simulink library "Nibble_Multiplexers_Lib"  (Simulink 8.7)
settings: Solver=ode45  StartTime=0.0  StopTime=10.0  RelTol=1e-3
libraries: Bit_Multiplexers_Lib x20, commutil2 x16
(part 1 of 2)
settings Model: Creator=uzivatel  LastModifiedBy=Jozko Mrkvicka

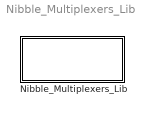
== system Nibble_Multiplexers_Lib ==
  Nibble_Multiplexers_Lib : Subsystem

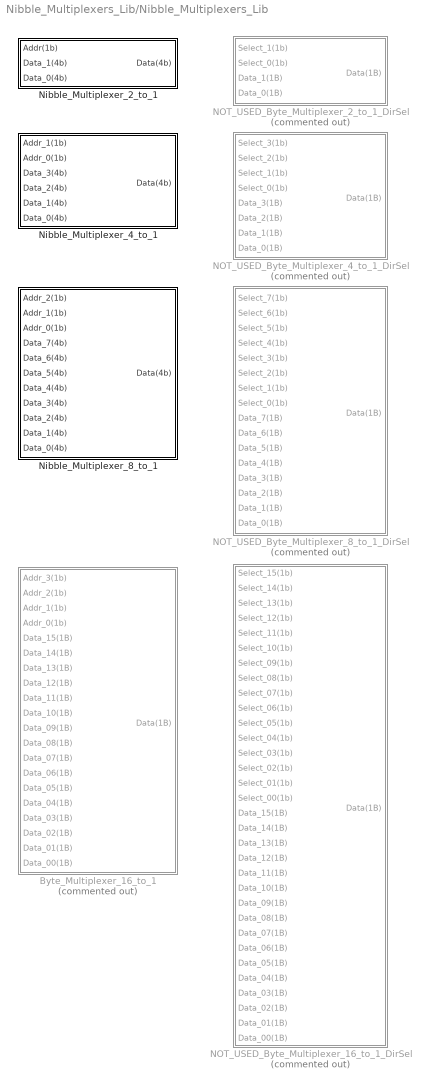
== system Nibble_Multiplexers_Lib/Nibble_Multiplexers_Lib ==
  Byte_Multiplexer_16_to_1 : Subsystem  Commented=on
  NOT_USED_Byte_Multiplexer_16_to_1_DirSel : Subsystem  Commented=on
  NOT_USED_Byte_Multiplexer_2_to_1_DirSel : Subsystem  Commented=on
  NOT_USED_Byte_Multiplexer_4_to_1_DirSel : Subsystem  Commented=on
  NOT_USED_Byte_Multiplexer_8_to_1_DirSel : Subsystem  Commented=on
  Nibble_Multiplexer_2_to_1 : Subsystem
  Nibble_Multiplexer_4_to_1 : Subsystem
  Nibble_Multiplexer_8_to_1 : Subsystem

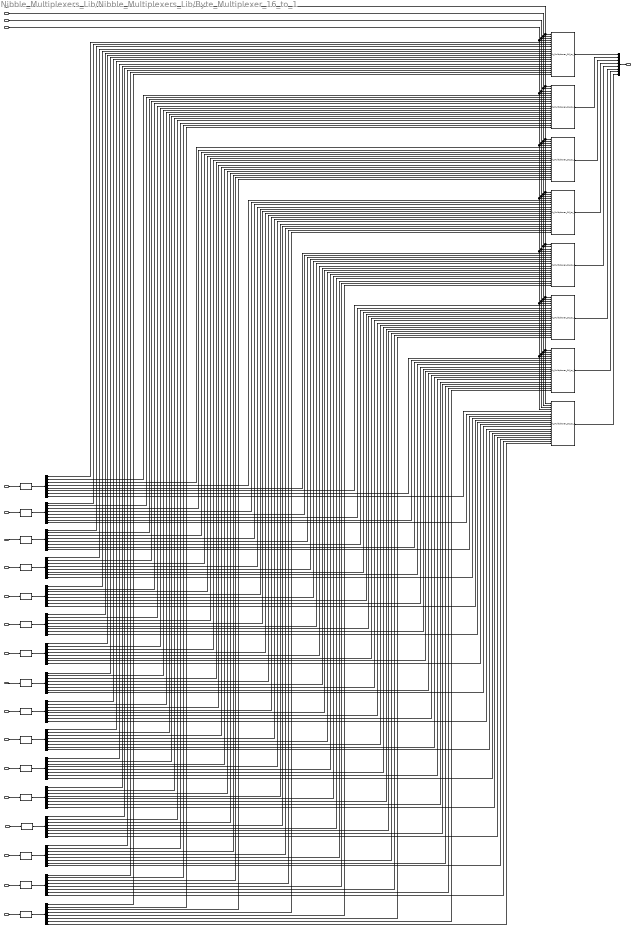
== system Nibble_Multiplexers_Lib/Nibble_Multiplexers_Lib/Byte_Multiplexer_16_to_1 ==
  Addr_3(1b) : Inport
  Addr_2(1b) : Inport  Port=2
  Addr_1(1b) : Inport  Port=3
  Addr_0(1b) : Inport  Port=4
  Data_15(1B) : Inport  Port=5
  Data_14(1B) : Inport  Port=6
  Data_13(1B) : Inport  Port=7
  Data_12(1B) : Inport  Port=8
  Data_11(1B) : Inport  Port=9
  Data_10(1B) : Inport  Port=10
  Data_09(1B) : Inport  Port=11
  Data_08(1B) : Inport  Port=12
  Data_07(1B) : Inport  Port=13
  Data_06(1B) : Inport  Port=14
  Data_05(1B) : Inport  Port=15
  Data_04(1B) : Inport  Port=16
  Data_03(1B) : Inport  Port=17
  Data_02(1B) : Inport  Port=18
  Data_01(1B) : Inport  Port=19
  Data_00(1B) : Inport  Port=20
  Bit_Multiplexer_16_to_1(Bit_0) : Bit_Multiplexers_Lib/Bit_Multiplexers_Lib/Bit_Multiplexer_16_to_1
  Bit_Multiplexer_16_to_1(Bit_1) : Bit_Multiplexers_Lib/Bit_Multiplexers_Lib/Bit_Multiplexer_16_to_1
  Bit_Multiplexer_16_to_1(Bit_2) : Bit_Multiplexers_Lib/Bit_Multiplexers_Lib/Bit_Multiplexer_16_to_1
  Bit_Multiplexer_16_to_1(Bit_3) : Bit_Multiplexers_Lib/Bit_Multiplexers_Lib/Bit_Multiplexer_16_to_1
  Bit_Multiplexer_16_to_1(Bit_4) : Bit_Multiplexers_Lib/Bit_Multiplexers_Lib/Bit_Multiplexer_16_to_1
  Bit_Multiplexer_16_to_1(Bit_5) : Bit_Multiplexers_Lib/Bit_Multiplexers_Lib/Bit_Multiplexer_16_to_1
  Bit_Multiplexer_16_to_1(Bit_6) : Bit_Multiplexers_Lib/Bit_Multiplexers_Lib/Bit_Multiplexer_16_to_1
  Bit_Multiplexer_16_to_1(Bit_7) : Bit_Multiplexers_Lib/Bit_Multiplexers_Lib/Bit_Multiplexer_16_to_1
  Bus Creator : BusCreator  Inputs=8
  Byte_{0..15} (16 alike) : Demux  Outputs=8
  Integer to Bit Converter{1..16} (16 alike) : commutil2/Integer to Bit Converter  nbits=8  signedInputValues=Unsigned  bitOrder=MSB first  outDtype=boolean
  Data(1B) : Outport
  wires:
  Integer to Bit Converter7/1 -> Byte_15/1
  Data_15(1B)/1 -> Integer to Bit Converter7/1
  Bus Creator/1 -> Data(1B)/1
  Addr_0(1b)/1 -> Bit_Multiplexer_16_to_1(Bit_5)/4, Bit_Multiplexer_16_to_1(Bit_0)/4, Bit_Multiplexer_16_to_1(Bit_1)/4, Bit_Multiplexer_16_to_1(Bit_2)/4, Bit_Multiplexer_16_to_1(Bit_3)/4, Bit_Multiplexer_16_to_1(Bit_4)/4, Bit_Multiplexer_16_to_1(Bit_6)/4, Bit_Multiplexer_16_to_1(Bit_7)/4
  Addr_1(1b)/1 -> Bit_Multiplexer_16_to_1(Bit_5)/3, Bit_Multiplexer_16_to_1(Bit_0)/3, Bit_Multiplexer_16_to_1(Bit_1)/3, Bit_Multiplexer_16_to_1(Bit_2)/3, Bit_Multiplexer_16_to_1(Bit_3)/3, Bit_Multiplexer_16_to_1(Bit_4)/3, Bit_Multiplexer_16_to_1(Bit_6)/3, Bit_Multiplexer_16_to_1(Bit_7)/3
  Addr_2(1b)/1 -> Bit_Multiplexer_16_to_1(Bit_6)/2, Bit_Multiplexer_16_to_1(Bit_5)/2, Bit_Multiplexer_16_to_1(Bit_4)/2, Bit_Multiplexer_16_to_1(Bit_2)/2, Bit_Multiplexer_16_to_1(Bit_1)/2, Bit_Multiplexer_16_to_1(Bit_0)/2, Bit_Multiplexer_16_to_1(Bit_3)/2, Bit_Multiplexer_16_to_1(Bit_7)/2
  Addr_3(1b)/1 -> Bit_Multiplexer_16_to_1(Bit_5)/1, Bit_Multiplexer_16_to_1(Bit_0)/1, Bit_Multiplexer_16_to_1(Bit_1)/1, Bit_Multiplexer_16_to_1(Bit_2)/1, Bit_Multiplexer_16_to_1(Bit_3)/1, Bit_Multiplexer_16_to_1(Bit_4)/1, Bit_Multiplexer_16_to_1(Bit_6)/1, Bit_Multiplexer_16_to_1(Bit_7)/1
  Bit_Multiplexer_16_to_1(Bit_4)/1 -> Bus Creator/4
  Bit_Multiplexer_16_to_1(Bit_5)/1 -> Bus Creator/3
  Bit_Multiplexer_16_to_1(Bit_6)/1 -> Bus Creator/2
  Bit_Multiplexer_16_to_1(Bit_7)/1 -> Bus Creator/1
  Bit_Multiplexer_16_to_1(Bit_3)/1 -> Bus Creator/5
  Bit_Multiplexer_16_to_1(Bit_2)/1 -> Bus Creator/6
  Bit_Multiplexer_16_to_1(Bit_1)/1 -> Bus Creator/7
  Bit_Multiplexer_16_to_1(Bit_0)/1 -> Bus Creator/8
  Integer to Bit Converter1/1 -> Byte_14/1
  Data_14(1B)/1 -> Integer to Bit Converter1/1
  Integer to Bit Converter2/1 -> Byte_13/1
  Data_13(1B)/1 -> Integer to Bit Converter2/1
  Integer to Bit Converter3/1 -> Byte_12/1
  Data_12(1B)/1 -> Integer to Bit Converter3/1
  Integer to Bit Converter4/1 -> Byte_11/1
  Data_11(1B)/1 -> Integer to Bit Converter4/1
  Integer to Bit Converter5/1 -> Byte_10/1
  Data_10(1B)/1 -> Integer to Bit Converter5/1
  Integer to Bit Converter6/1 -> Byte_9/1
  Data_09(1B)/1 -> Integer to Bit Converter6/1
  Integer to Bit Converter8/1 -> Byte_8/1
  Data_08(1B)/1 -> Integer to Bit Converter8/1
  Integer to Bit Converter9/1 -> Byte_7/1
  Data_07(1B)/1 -> Integer to Bit Converter9/1
  Integer to Bit Converter10/1 -> Byte_6/1
  Data_06(1B)/1 -> Integer to Bit Converter10/1
  Integer to Bit Converter11/1 -> Byte_5/1
  Data_05(1B)/1 -> Integer to Bit Converter11/1
  Integer to Bit Converter12/1 -> Byte_4/1
  Data_04(1B)/1 -> Integer to Bit Converter12/1
  Integer to Bit Converter13/1 -> Byte_3/1
  Data_03(1B)/1 -> Integer to Bit Converter13/1
  Integer to Bit Converter14/1 -> Byte_2/1
  Data_02(1B)/1 -> Integer to Bit Converter14/1
  Integer to Bit Converter15/1 -> Byte_1/1
  Data_01(1B)/1 -> Integer to Bit Converter15/1
  Integer to Bit Converter16/1 -> Byte_0/1
  Data_00(1B)/1 -> Integer to Bit Converter16/1
  Byte_15/1 -> Bit_Multiplexer_16_to_1(Bit_7)/5
  Byte_14/1 -> Bit_Multiplexer_16_to_1(Bit_7)/6
  Byte_13/1 -> Bit_Multiplexer_16_to_1(Bit_7)/7
  Byte_12/1 -> Bit_Multiplexer_16_to_1(Bit_7)/8
  Byte_11/1 -> Bit_Multiplexer_16_to_1(Bit_7)/9
  Byte_10/1 -> Bit_Multiplexer_16_to_1(Bit_7)/10
  Byte_9/1 -> Bit_Multiplexer_16_to_1(Bit_7)/11
  Byte_8/1 -> Bit_Multiplexer_16_to_1(Bit_7)/12
  Byte_7/1 -> Bit_Multiplexer_16_to_1(Bit_7)/13
  Byte_6/1 -> Bit_Multiplexer_16_to_1(Bit_7)/14
  Byte_5/1 -> Bit_Multiplexer_16_to_1(Bit_7)/15
  Byte_4/1 -> Bit_Multiplexer_16_to_1(Bit_7)/16
  Byte_3/1 -> Bit_Multiplexer_16_to_1(Bit_7)/17
  Byte_2/1 -> Bit_Multiplexer_16_to_1(Bit_7)/18
  Byte_1/1 -> Bit_Multiplexer_16_to_1(Bit_7)/19
  Byte_0/1 -> Bit_Multiplexer_16_to_1(Bit_7)/20
  Byte_15/2 -> Bit_Multiplexer_16_to_1(Bit_6)/5
  Byte_14/2 -> Bit_Multiplexer_16_to_1(Bit_6)/6
  Byte_13/2 -> Bit_Multiplexer_16_to_1(Bit_6)/7
  Byte_12/2 -> Bit_Multiplexer_16_to_1(Bit_6)/8
  Byte_11/2 -> Bit_Multiplexer_16_to_1(Bit_6)/9
  Byte_10/2 -> Bit_Multiplexer_16_to_1(Bit_6)/10
  Byte_9/2 -> Bit_Multiplexer_16_to_1(Bit_6)/11
  Byte_8/2 -> Bit_Multiplexer_16_to_1(Bit_6)/12
  Byte_7/2 -> Bit_Multiplexer_16_to_1(Bit_6)/13
  Byte_6/2 -> Bit_Multiplexer_16_to_1(Bit_6)/14
  Byte_5/2 -> Bit_Multiplexer_16_to_1(Bit_6)/15
  Byte_4/2 -> Bit_Multiplexer_16_to_1(Bit_6)/16
  Byte_3/2 -> Bit_Multiplexer_16_to_1(Bit_6)/17
  Byte_2/2 -> Bit_Multiplexer_16_to_1(Bit_6)/18
  Byte_1/2 -> Bit_Multiplexer_16_to_1(Bit_6)/19
  Byte_0/2 -> Bit_Multiplexer_16_to_1(Bit_6)/20
  Byte_15/3 -> Bit_Multiplexer_16_to_1(Bit_5)/5
  Byte_14/3 -> Bit_Multiplexer_16_to_1(Bit_5)/6
  Byte_13/3 -> Bit_Multiplexer_16_to_1(Bit_5)/7
  Byte_12/3 -> Bit_Multiplexer_16_to_1(Bit_5)/8
  Byte_11/3 -> Bit_Multiplexer_16_to_1(Bit_5)/9
  Byte_10/3 -> Bit_Multiplexer_16_to_1(Bit_5)/10
  Byte_9/3 -> Bit_Multiplexer_16_to_1(Bit_5)/11
  Byte_8/3 -> Bit_Multiplexer_16_to_1(Bit_5)/12
  Byte_7/3 -> Bit_Multiplexer_16_to_1(Bit_5)/13
  Byte_6/3 -> Bit_Multiplexer_16_to_1(Bit_5)/14
  Byte_5/3 -> Bit_Multiplexer_16_to_1(Bit_5)/15
  Byte_4/3 -> Bit_Multiplexer_16_to_1(Bit_5)/16
  Byte_3/3 -> Bit_Multiplexer_16_to_1(Bit_5)/17
  Byte_2/3 -> Bit_Multiplexer_16_to_1(Bit_5)/18
  Byte_1/3 -> Bit_Multiplexer_16_to_1(Bit_5)/19
  Byte_0/3 -> Bit_Multiplexer_16_to_1(Bit_5)/20
  Byte_15/4 -> Bit_Multiplexer_16_to_1(Bit_4)/5
  Byte_14/4 -> Bit_Multiplexer_16_to_1(Bit_4)/6
  Byte_13/4 -> Bit_Multiplexer_16_to_1(Bit_4)/7
  Byte_12/4 -> Bit_Multiplexer_16_to_1(Bit_4)/8
  Byte_11/4 -> Bit_Multiplexer_16_to_1(Bit_4)/9
  Byte_10/4 -> Bit_Multiplexer_16_to_1(Bit_4)/10
  Byte_9/4 -> Bit_Multiplexer_16_to_1(Bit_4)/11
  Byte_8/4 -> Bit_Multiplexer_16_to_1(Bit_4)/12
  Byte_7/4 -> Bit_Multiplexer_16_to_1(Bit_4)/13
  Byte_6/4 -> Bit_Multiplexer_16_to_1(Bit_4)/14
  Byte_5/4 -> Bit_Multiplexer_16_to_1(Bit_4)/15
  Byte_4/4 -> Bit_Multiplexer_16_to_1(Bit_4)/16
  Byte_3/4 -> Bit_Multiplexer_16_to_1(Bit_4)/17
  Byte_2/4 -> Bit_Multiplexer_16_to_1(Bit_4)/18
  Byte_1/4 -> Bit_Multiplexer_16_to_1(Bit_4)/19
  Byte_0/4 -> Bit_Multiplexer_16_to_1(Bit_4)/20
  Byte_15/5 -> Bit_Multiplexer_16_to_1(Bit_3)/5
  Byte_14/5 -> Bit_Multiplexer_16_to_1(Bit_3)/6
  Byte_13/5 -> Bit_Multiplexer_16_to_1(Bit_3)/7
  Byte_12/5 -> Bit_Multiplexer_16_to_1(Bit_3)/8
  Byte_11/5 -> Bit_Multiplexer_16_to_1(Bit_3)/9
  Byte_10/5 -> Bit_Multiplexer_16_to_1(Bit_3)/10
  Byte_9/5 -> Bit_Multiplexer_16_to_1(Bit_3)/11
  Byte_8/5 -> Bit_Multiplexer_16_to_1(Bit_3)/12
  Byte_7/5 -> Bit_Multiplexer_16_to_1(Bit_3)/13
  Byte_6/5 -> Bit_Multiplexer_16_to_1(Bit_3)/14
  Byte_5/5 -> Bit_Multiplexer_16_to_1(Bit_3)/15
  Byte_4/5 -> Bit_Multiplexer_16_to_1(Bit_3)/16
  Byte_3/5 -> Bit_Multiplexer_16_to_1(Bit_3)/17
  Byte_2/5 -> Bit_Multiplexer_16_to_1(Bit_3)/18
  Byte_1/5 -> Bit_Multiplexer_16_to_1(Bit_3)/19
  Byte_0/5 -> Bit_Multiplexer_16_to_1(Bit_3)/20
  Byte_15/6 -> Bit_Multiplexer_16_to_1(Bit_2)/5
  Byte_14/6 -> Bit_Multiplexer_16_to_1(Bit_2)/6
  Byte_13/6 -> Bit_Multiplexer_16_to_1(Bit_2)/7
  Byte_12/6 -> Bit_Multiplexer_16_to_1(Bit_2)/8
  Byte_11/6 -> Bit_Multiplexer_16_to_1(Bit_2)/9
  Byte_10/6 -> Bit_Multiplexer_16_to_1(Bit_2)/10
  Byte_9/6 -> Bit_Multiplexer_16_to_1(Bit_2)/11
  Byte_8/6 -> Bit_Multiplexer_16_to_1(Bit_2)/12
  Byte_7/6 -> Bit_Multiplexer_16_to_1(Bit_2)/13
  Byte_6/6 -> Bit_Multiplexer_16_to_1(Bit_2)/14
  Byte_5/6 -> Bit_Multiplexer_16_to_1(Bit_2)/15
  Byte_4/6 -> Bit_Multiplexer_16_to_1(Bit_2)/16
  Byte_3/6 -> Bit_Multiplexer_16_to_1(Bit_2)/17
  Byte_2/6 -> Bit_Multiplexer_16_to_1(Bit_2)/18
  Byte_1/6 -> Bit_Multiplexer_16_to_1(Bit_2)/19
  Byte_0/6 -> Bit_Multiplexer_16_to_1(Bit_2)/20
  Byte_15/7 -> Bit_Multiplexer_16_to_1(Bit_1)/5
  Byte_14/7 -> Bit_Multiplexer_16_to_1(Bit_1)/6
  Byte_13/7 -> Bit_Multiplexer_16_to_1(Bit_1)/7
  Byte_12/7 -> Bit_Multiplexer_16_to_1(Bit_1)/8
  Byte_11/7 -> Bit_Multiplexer_16_to_1(Bit_1)/9
  Byte_10/7 -> Bit_Multiplexer_16_to_1(Bit_1)/10
  Byte_9/7 -> Bit_Multiplexer_16_to_1(Bit_1)/11
  Byte_8/7 -> Bit_Multiplexer_16_to_1(Bit_1)/12
  Byte_7/7 -> Bit_Multiplexer_16_to_1(Bit_1)/13
  Byte_6/7 -> Bit_Multiplexer_16_to_1(Bit_1)/14
  Byte_5/7 -> Bit_Multiplexer_16_to_1(Bit_1)/15
  Byte_4/7 -> Bit_Multiplexer_16_to_1(Bit_1)/16
  Byte_3/7 -> Bit_Multiplexer_16_to_1(Bit_1)/17
  Byte_2/7 -> Bit_Multiplexer_16_to_1(Bit_1)/18
  Byte_1/7 -> Bit_Multiplexer_16_to_1(Bit_1)/19
  Byte_0/7 -> Bit_Multiplexer_16_to_1(Bit_1)/20
  Byte_15/8 -> Bit_Multiplexer_16_to_1(Bit_0)/5
  Byte_14/8 -> Bit_Multiplexer_16_to_1(Bit_0)/6
  Byte_13/8 -> Bit_Multiplexer_16_to_1(Bit_0)/7
  Byte_12/8 -> Bit_Multiplexer_16_to_1(Bit_0)/8
  Byte_11/8 -> Bit_Multiplexer_16_to_1(Bit_0)/9
  Byte_10/8 -> Bit_Multiplexer_16_to_1(Bit_0)/10
  Byte_9/8 -> Bit_Multiplexer_16_to_1(Bit_0)/11
  Byte_8/8 -> Bit_Multiplexer_16_to_1(Bit_0)/12
  Byte_7/8 -> Bit_Multiplexer_16_to_1(Bit_0)/13
  Byte_6/8 -> Bit_Multiplexer_16_to_1(Bit_0)/14
  Byte_5/8 -> Bit_Multiplexer_16_to_1(Bit_0)/15
  Byte_4/8 -> Bit_Multiplexer_16_to_1(Bit_0)/16
  Byte_3/8 -> Bit_Multiplexer_16_to_1(Bit_0)/17
  Byte_2/8 -> Bit_Multiplexer_16_to_1(Bit_0)/18
  Byte_1/8 -> Bit_Multiplexer_16_to_1(Bit_0)/19
  Byte_0/8 -> Bit_Multiplexer_16_to_1(Bit_0)/20

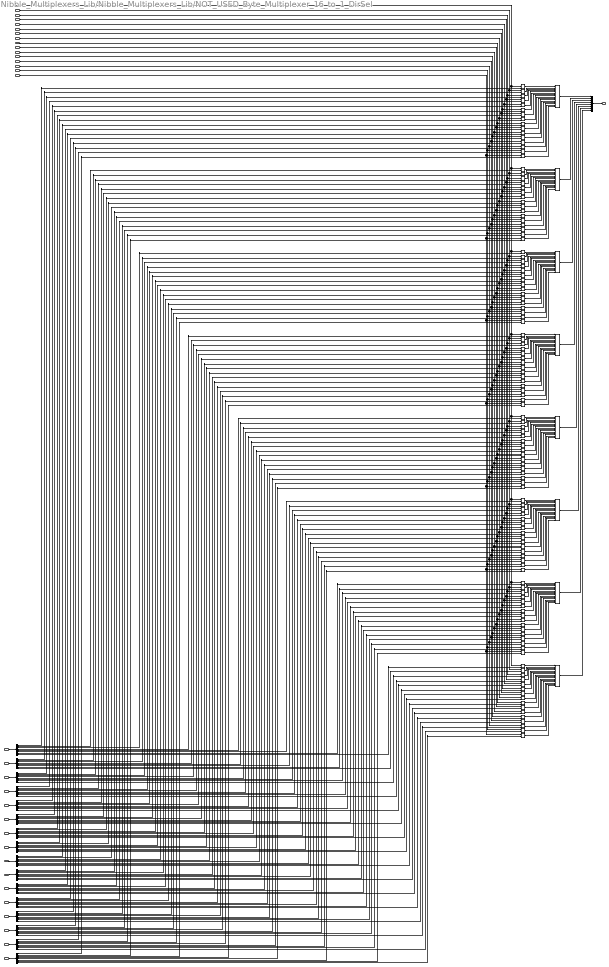
== system Nibble_Multiplexers_Lib/Nibble_Multiplexers_Lib/NOT_USED_Byte_Multiplexer_16_to_1_DirSel ==
  note: Bit_Multiplexer_16_to_1_DirSel(Bit_07)
  note: Bit_Multiplexer_16_to_1_DirSel(Bit_06)
  note: Bit_Multiplexer_16_to_1_DirSel(Bit_05)
  note: Bit_Multiplexer_16_to_1_DirSel(Bit_04)
  note: Bit_Multiplexer_16_to_1_DirSel(Bit_03)
  note: Bit_Multiplexer_16_to_1_DirSel(Bit_02)
  note: Bit_Multiplexer_16_to_1_DirSel(Bit_01)
  note: Bit_Multiplexer_16_to_1_DirSel(Bit_00)
  Select_15(1b) : Inport
  Select_14(1b) : Inport  Port=2
  Select_13(1b) : Inport  Port=3
  Select_12(1b) : Inport  Port=4
  Select_11(1b) : Inport  Port=5
  Select_10(1b) : Inport  Port=6
  Select_09(1b) : Inport  Port=7
  Select_08(1b) : Inport  Port=8
  Select_07(1b) : Inport  Port=9
  Select_06(1b) : Inport  Port=10
  Select_05(1b) : Inport  Port=11
  Select_04(1b) : Inport  Port=12
  Select_03(1b) : Inport  Port=13
  Select_02(1b) : Inport  Port=14
  Select_01(1b) : Inport  Port=15
  Select_00(1b) : Inport  Port=16
  Data_15(1B) : Inport  Port=17
  Data_14(1B) : Inport  Port=18
  Data_13(1B) : Inport  Port=19
  Data_12(1B) : Inport  Port=20
  Data_11(1B) : Inport  Port=21
  Data_10(1B) : Inport  Port=22
  Data_09(1B) : Inport  Port=23
  Data_08(1B) : Inport  Port=24
  Data_07(1B) : Inport  Port=25
  Data_06(1B) : Inport  Port=26
  Data_05(1B) : Inport  Port=27
  Data_04(1B) : Inport  Port=28
  Data_03(1B) : Inport  Port=29
  Data_02(1B) : Inport  Port=30
  Data_01(1B) : Inport  Port=31
  Data_00(1B) : Inport  Port=32
  Bus Creator : BusCreator  Inputs=8
  Bus Selector{1..16} (16 alike) : BusSelector  OutputSignals=signal1,signal2,signal3,signal4,signal5,signal6,signal7,signal8
  Logical Operator{137..151,153..168,170..185,187..202,204..219,221..236,238..253,255..270,272} (128 alike) : Logic  IconShape=distinctive  AllPortsSameDT=off  OutDataTypeStr=boolean
  Logical Operator{152,169,186,203,220,237,254,271} (8 alike) : Logic  Operator=OR  Inputs=16  IconShape=distinctive  OutDataTypeStr=boolean
  Data(1B) : Outport
  wires:
  Data_15(1B)/1 -> Bus Selector15/1
  Data_14(1B)/1 -> Bus Selector1/1
  Data_13(1B)/1 -> Bus Selector2/1
  Data_12(1B)/1 -> Bus Selector3/1
  Data_11(1B)/1 -> Bus Selector4/1
  Data_10(1B)/1 -> Bus Selector5/1
  Data_09(1B)/1 -> Bus Selector6/1
  Data_08(1B)/1 -> Bus Selector7/1
  Data_07(1B)/1 -> Bus Selector8/1
  Data_06(1B)/1 -> Bus Selector9/1
  Data_05(1B)/1 -> Bus Selector10/1
  Data_04(1B)/1 -> Bus Selector11/1
  Data_03(1B)/1 -> Bus Selector12/1
  Data_02(1B)/1 -> Bus Selector13/1
  Data_01(1B)/1 -> Bus Selector14/1
  Data_00(1B)/1 -> Bus Selector16/1
  Bus Creator/1 -> Data(1B)/1
  Bus Selector16/8 -> Logical Operator264/2  "<signal8>"
  Bus Selector14/8 -> Logical Operator263/2  "<signal8>"
  Bus Selector13/8 -> Logical Operator262/2  "<signal8>"
  Bus Selector12/8 -> Logical Operator261/2  "<signal8>"
  Bus Selector11/8 -> Logical Operator258/2  "<signal8>"
  Bus Selector10/8 -> Logical Operator257/2  "<signal8>"
  Bus Selector9/8 -> Logical Operator256/2  "<signal8>"
  Bus Selector8/8 -> Logical Operator272/2  "<signal8>"
  Bus Selector15/8 -> Logical Operator259/2  "<signal8>"
  Bus Selector1/8 -> Logical Operator260/2  "<signal8>"
  Bus Selector2/8 -> Logical Operator265/2  "<signal8>"
  Bus Selector3/8 -> Logical Operator266/2  "<signal8>"
  Bus Selector4/8 -> Logical Operator267/2  "<signal8>"
  Bus Selector5/8 -> Logical Operator268/2  "<signal8>"
  Bus Selector6/8 -> Logical Operator269/2  "<signal8>"
  Bus Selector7/8 -> Logical Operator270/2  "<signal8>"
  Bus Selector16/7 -> Logical Operator247/2  "<signal7>"
  Bus Selector14/7 -> Logical Operator246/2  "<signal7>"
  Bus Selector13/7 -> Logical Operator245/2  "<signal7>"
  Bus Selector12/7 -> Logical Operator244/2  "<signal7>"
  Bus Selector11/7 -> Logical Operator241/2  "<signal7>"
  Bus Selector10/7 -> Logical Operator240/2  "<signal7>"
  Bus Selector9/7 -> Logical Operator239/2  "<signal7>"
  Bus Selector8/7 -> Logical Operator255/2  "<signal7>"
  Bus Selector15/7 -> Logical Operator242/2  "<signal7>"
  Bus Selector1/7 -> Logical Operator243/2  "<signal7>"
  Bus Selector2/7 -> Logical Operator248/2  "<signal7>"
  Bus Selector3/7 -> Logical Operator249/2  "<signal7>"
  Bus Selector4/7 -> Logical Operator250/2  "<signal7>"
  Bus Selector5/7 -> Logical Operator251/2  "<signal7>"
  Bus Selector6/7 -> Logical Operator252/2  "<signal7>"
  Bus Selector7/7 -> Logical Operator253/2  "<signal7>"
  Bus Selector16/6 -> Logical Operator230/2  "<signal6>"
  Bus Selector14/6 -> Logical Operator229/2  "<signal6>"
  Bus Selector13/6 -> Logical Operator228/2  "<signal6>"
  Bus Selector12/6 -> Logical Operator227/2  "<signal6>"
  Bus Selector11/6 -> Logical Operator224/2  "<signal6>"
  Bus Selector10/6 -> Logical Operator223/2  "<signal6>"
  Bus Selector9/6 -> Logical Operator222/2  "<signal6>"
  Bus Selector8/6 -> Logical Operator238/2  "<signal6>"
  Bus Selector15/6 -> Logical Operator225/2  "<signal6>"
  Bus Selector1/6 -> Logical Operator226/2  "<signal6>"
  Bus Selector2/6 -> Logical Operator231/2  "<signal6>"
  Bus Selector3/6 -> Logical Operator232/2  "<signal6>"
  Bus Selector4/6 -> Logical Operator233/2  "<signal6>"
  Bus Selector5/6 -> Logical Operator234/2  "<signal6>"
  Bus Selector6/6 -> Logical Operator235/2  "<signal6>"
  Bus Selector7/6 -> Logical Operator236/2  "<signal6>"
  Bus Selector16/5 -> Logical Operator213/2  "<signal5>"
  Bus Selector14/5 -> Logical Operator212/2  "<signal5>"
  Bus Selector13/5 -> Logical Operator211/2  "<signal5>"
  Bus Selector12/5 -> Logical Operator210/2  "<signal5>"
  Bus Selector11/5 -> Logical Operator207/2  "<signal5>"
  Bus Selector10/5 -> Logical Operator206/2  "<signal5>"
  Bus Selector9/5 -> Logical Operator205/2  "<signal5>"
  Bus Selector8/5 -> Logical Operator221/2  "<signal5>"
  Bus Selector15/5 -> Logical Operator208/2  "<signal5>"
  Bus Selector1/5 -> Logical Operator209/2  "<signal5>"
  Bus Selector2/5 -> Logical Operator214/2  "<signal5>"
  Bus Selector3/5 -> Logical Operator215/2  "<signal5>"
  Bus Selector4/5 -> Logical Operator216/2  "<signal5>"
  Bus Selector5/5 -> Logical Operator217/2  "<signal5>"
  Bus Selector6/5 -> Logical Operator218/2  "<signal5>"
  Bus Selector7/5 -> Logical Operator219/2  "<signal5>"
  Bus Selector16/4 -> Logical Operator196/2  "<signal4>"
  Bus Selector14/4 -> Logical Operator195/2  "<signal4>"
  Bus Selector13/4 -> Logical Operator194/2  "<signal4>"
  Bus Selector12/4 -> Logical Operator193/2  "<signal4>"
  Bus Selector11/4 -> Logical Operator190/2  "<signal4>"
  Bus Selector10/4 -> Logical Operator189/2  "<signal4>"
  Bus Selector9/4 -> Logical Operator188/2  "<signal4>"
  Bus Selector8/4 -> Logical Operator204/2  "<signal4>"
  Bus Selector15/4 -> Logical Operator191/2  "<signal4>"
  Bus Selector1/4 -> Logical Operator192/2  "<signal4>"
  Bus Selector2/4 -> Logical Operator197/2  "<signal4>"
  Bus Selector3/4 -> Logical Operator198/2  "<signal4>"
  Bus Selector4/4 -> Logical Operator199/2  "<signal4>"
  Bus Selector5/4 -> Logical Operator200/2  "<signal4>"
  Bus Selector6/4 -> Logical Operator201/2  "<signal4>"
  Bus Selector7/4 -> Logical Operator202/2  "<signal4>"
  Bus Selector16/3 -> Logical Operator179/2  "<signal3>"
  Bus Selector14/3 -> Logical Operator178/2  "<signal3>"
  Bus Selector13/3 -> Logical Operator177/2  "<signal3>"
  Bus Selector12/3 -> Logical Operator176/2  "<signal3>"
  Bus Selector11/3 -> Logical Operator173/2  "<signal3>"
  Bus Selector10/3 -> Logical Operator172/2  "<signal3>"
  Bus Selector9/3 -> Logical Operator171/2  "<signal3>"
  Bus Selector8/3 -> Logical Operator187/2  "<signal3>"
  Bus Selector15/3 -> Logical Operator174/2  "<signal3>"
  Bus Selector1/3 -> Logical Operator175/2  "<signal3>"
  Bus Selector2/3 -> Logical Operator180/2  "<signal3>"
  Bus Selector3/3 -> Logical Operator181/2  "<signal3>"
  Bus Selector4/3 -> Logical Operator182/2  "<signal3>"
  Bus Selector5/3 -> Logical Operator183/2  "<signal3>"
  Bus Selector6/3 -> Logical Operator184/2  "<signal3>"
  Bus Selector7/3 -> Logical Operator185/2  "<signal3>"
  Bus Selector16/2 -> Logical Operator162/2  "<signal2>"
  Bus Selector14/2 -> Logical Operator161/2  "<signal2>"
  Bus Selector13/2 -> Logical Operator160/2  "<signal2>"
  Bus Selector12/2 -> Logical Operator159/2  "<signal2>"
  Bus Selector11/2 -> Logical Operator156/2  "<signal2>"
  Bus Selector10/2 -> Logical Operator155/2  "<signal2>"
  Bus Selector9/2 -> Logical Operator154/2  "<signal2>"
  Bus Selector8/2 -> Logical Operator170/2  "<signal2>"
  Bus Selector15/2 -> Logical Operator157/2  "<signal2>"
  Bus Selector1/2 -> Logical Operator158/2  "<signal2>"
  Bus Selector2/2 -> Logical Operator163/2  "<signal2>"
  Bus Selector3/2 -> Logical Operator164/2  "<signal2>"
  Bus Selector4/2 -> Logical Operator165/2  "<signal2>"
  Bus Selector5/2 -> Logical Operator166/2  "<signal2>"
  Bus Selector6/2 -> Logical Operator167/2  "<signal2>"
  Bus Selector7/2 -> Logical Operator168/2  "<signal2>"
  Bus Selector16/1 -> Logical Operator145/2  "<signal1>"
  Bus Selector14/1 -> Logical Operator144/2  "<signal1>"
  Bus Selector13/1 -> Logical Operator143/2  "<signal1>"
  Bus Selector12/1 -> Logical Operator142/2  "<signal1>"
  Bus Selector11/1 -> Logical Operator139/2  "<signal1>"
  Bus Selector10/1 -> Logical Operator138/2  "<signal1>"
  Bus Selector9/1 -> Logical Operator137/2  "<signal1>"
  Bus Selector8/1 -> Logical Operator153/2  "<signal1>"
  Bus Selector15/1 -> Logical Operator140/2  "<signal1>"
  Bus Selector1/1 -> Logical Operator141/2  "<signal1>"
  Bus Selector2/1 -> Logical Operator146/2  "<signal1>"
  Bus Selector3/1 -> Logical Operator147/2  "<signal1>"
  Bus Selector4/1 -> Logical Operator148/2  "<signal1>"
  Bus Selector5/1 -> Logical Operator149/2  "<signal1>"
  Bus Selector6/1 -> Logical Operator150/2  "<signal1>"
  Bus Selector7/1 -> Logical Operator151/2  "<signal1>"
  Select_15(1b)/1 -> Logical Operator225/1, Logical Operator259/1, Logical Operator242/1, Logical Operator208/1, Logical Operator191/1, Logical Operator174/1, Logical Operator157/1, Logical Operator140/1
  Select_14(1b)/1 -> Logical Operator260/1, Logical Operator243/1, Logical Operator226/1, Logical Operator209/1, Logical Operator192/1, Logical Operator175/1, Logical Operator158/1, Logical Operator141/1
  Select_13(1b)/1 -> Logical Operator265/1, Logical Operator248/1, Logical Operator231/1, Logical Operator214/1, Logical Operator197/1, Logical Operator180/1, Logical Operator163/1, Logical Operator146/1
  Select_12(1b)/1 -> Logical Operator266/1, Logical Operator249/1, Logical Operator232/1, Logical Operator215/1, Logical Operator198/1, Logical Operator181/1, Logical Operator164/1, Logical Operator147/1
  Select_11(1b)/1 -> Logical Operator267/1, Logical Operator250/1, Logical Operator233/1, Logical Operator216/1, Logical Operator199/1, Logical Operator182/1, Logical Operator165/1, Logical Operator148/1
  Select_10(1b)/1 -> Logical Operator268/1, Logical Operator251/1, Logical Operator234/1, Logical Operator217/1, Logical Operator200/1, Logical Operator183/1, Logical Operator166/1, Logical Operator149/1
  Select_09(1b)/1 -> Logical Operator269/1, Logical Operator252/1, Logical Operator235/1, Logical Operator218/1, Logical Operator201/1, Logical Operator184/1, Logical Operator167/1, Logical Operator150/1
  Select_08(1b)/1 -> Logical Operator270/1, Logical Operator253/1, Logical Operator236/1, Logical Operator219/1, Logical Operator202/1, Logical Operator185/1, Logical Operator168/1, Logical Operator151/1
  Select_07(1b)/1 -> Logical Operator272/1, Logical Operator255/1, Logical Operator238/1, Logical Operator221/1, Logical Operator204/1, Logical Operator187/1, Logical Operator170/1, Logical Operator153/1
  Select_06(1b)/1 -> Logical Operator256/1, Logical Operator239/1, Logical Operator222/1, Logical Operator205/1, Logical Operator188/1, Logical Operator171/1, Logical Operator154/1, Logical Operator137/1
  Select_04(1b)/1 -> Logical Operator258/1, Logical Operator241/1, Logical Operator224/1, Logical Operator207/1, Logical Operator190/1, Logical Operator173/1, Logical Operator156/1, Logical Operator139/1
  Select_03(1b)/1 -> Logical Operator261/1, Logical Operator244/1, Logical Operator227/1, Logical Operator210/1, Logical Operator193/1, Logical Operator176/1, Logical Operator159/1, Logical Operator142/1
  Select_02(1b)/1 -> Logical Operator262/1, Logical Operator245/1, Logical Operator228/1, Logical Operator211/1, Logical Operator194/1, Logical Operator177/1, Logical Operator160/1, Logical Operator143/1
  Select_00(1b)/1 -> Logical Operator264/1, Logical Operator247/1, Logical Operator230/1, Logical Operator213/1, Logical Operator196/1, Logical Operator179/1, Logical Operator162/1, Logical Operator145/1
  Logical Operator147/1 -> Logical Operator152/4
  Logical Operator146/1 -> Logical Operator152/3
  Logical Operator141/1 -> Logical Operator152/2
  Logical Operator140/1 -> Logical Operator152/1
  Logical Operator151/1 -> Logical Operator152/8
  Logical Operator150/1 -> Logical Operator152/7
  Logical Operator149/1 -> Logical Operator152/6
  Logical Operator148/1 -> Logical Operator152/5
  Logical Operator139/1 -> Logical Operator152/12
  Logical Operator138/1 -> Logical Operator152/11
  Logical Operator137/1 -> Logical Operator152/10
  Logical Operator153/1 -> Logical Operator152/9
  Logical Operator145/1 -> Logical Operator152/16
  Logical Operator144/1 -> Logical Operator152/15
  Logical Operator143/1 -> Logical Operator152/14
  Logical Operator142/1 -> Logical Operator152/13
  Logical Operator169/1 -> Bus Creator/2
  Logical Operator164/1 -> Logical Operator169/4
  Logical Operator163/1 -> Logical Operator169/3
  Logical Operator158/1 -> Logical Operator169/2
  Logical Operator157/1 -> Logical Operator169/1
  Logical Operator168/1 -> Logical Operator169/8
  Logical Operator167/1 -> Logical Operator169/7
  Logical Operator166/1 -> Logical Operator169/6
  Logical Operator165/1 -> Logical Operator169/5
  Logical Operator156/1 -> Logical Operator169/12
  Logical Operator155/1 -> Logical Operator169/11
  Logical Operator154/1 -> Logical Operator169/10
  Logical Operator170/1 -> Logical Operator169/9
  Logical Operator162/1 -> Logical Operator169/16
  Logical Operator161/1 -> Logical Operator169/15
  Logical Operator160/1 -> Logical Operator169/14
  Logical Operator159/1 -> Logical Operator169/13
  Logical Operator181/1 -> Logical Operator186/4
  Logical Operator180/1 -> Logical Operator186/3
  Logical Operator175/1 -> Logical Operator186/2
  Logical Operator174/1 -> Logical Operator186/1
  Logical Operator185/1 -> Logical Operator186/8
  Logical Operator184/1 -> Logical Operator186/7
  Logical Operator183/1 -> Logical Operator186/6
  Logical Operator182/1 -> Logical Operator186/5
  Logical Operator173/1 -> Logical Operator186/12
  Logical Operator172/1 -> Logical Operator186/11
  Logical Operator171/1 -> Logical Operator186/10
  Logical Operator187/1 -> Logical Operator186/9
  Logical Operator179/1 -> Logical Operator186/16
  Logical Operator178/1 -> Logical Operator186/15
  Logical Operator177/1 -> Logical Operator186/14
  Logical Operator176/1 -> Logical Operator186/13
  Logical Operator203/1 -> Bus Creator/4
  Logical Operator198/1 -> Logical Operator203/4
  Logical Operator197/1 -> Logical Operator203/3
  Logical Operator192/1 -> Logical Operator203/2
  Logical Operator191/1 -> Logical Operator203/1
  Logical Operator202/1 -> Logical Operator203/8
  Logical Operator201/1 -> Logical Operator203/7
  Logical Operator200/1 -> Logical Operator203/6
  Logical Operator199/1 -> Logical Operator203/5
  Logical Operator190/1 -> Logical Operator203/12
  Logical Operator189/1 -> Logical Operator203/11
  Logical Operator188/1 -> Logical Operator203/10
  Logical Operator204/1 -> Logical Operator203/9
  Logical Operator196/1 -> Logical Operator203/16
  Logical Operator195/1 -> Logical Operator203/15
  Logical Operator194/1 -> Logical Operator203/14
  Logical Operator193/1 -> Logical Operator203/13
  Logical Operator215/1 -> Logical Operator220/4
  Logical Operator214/1 -> Logical Operator220/3
  Logical Operator209/1 -> Logical Operator220/2
  Logical Operator208/1 -> Logical Operator220/1
  Logical Operator219/1 -> Logical Operator220/8
  Logical Operator218/1 -> Logical Operator220/7
  Logical Operator217/1 -> Logical Operator220/6
  Logical Operator216/1 -> Logical Operator220/5
  Logical Operator207/1 -> Logical Operator220/12
  Logical Operator206/1 -> Logical Operator220/11
  Logical Operator205/1 -> Logical Operator220/10
  Logical Operator221/1 -> Logical Operator220/9
  Logical Operator213/1 -> Logical Operator220/16
  Logical Operator212/1 -> Logical Operator220/15
  Logical Operator211/1 -> Logical Operator220/14
  Logical Operator210/1 -> Logical Operator220/13
  Logical Operator237/1 -> Bus Creator/6
  Logical Operator232/1 -> Logical Operator237/4
  Logical Operator231/1 -> Logical Operator237/3
  Logical Operator226/1 -> Logical Operator237/2
  Logical Operator225/1 -> Logical Operator237/1
  Logical Operator236/1 -> Logical Operator237/8
  Logical Operator235/1 -> Logical Operator237/7
  Logical Operator234/1 -> Logical Operator237/6
  Logical Operator233/1 -> Logical Operator237/5
  Logical Operator224/1 -> Logical Operator237/12
  Logical Operator223/1 -> Logical Operator237/11
  Logical Operator222/1 -> Logical Operator237/10
  Logical Operator238/1 -> Logical Operator237/9
  Logical Operator230/1 -> Logical Operator237/16
  Logical Operator229/1 -> Logical Operator237/15
  Logical Operator228/1 -> Logical Operator237/14
  Logical Operator227/1 -> Logical Operator237/13
  Logical Operator249/1 -> Logical Operator254/4
  Logical Operator248/1 -> Logical Operator254/3
  Logical Operator243/1 -> Logical Operator254/2
  Logical Operator242/1 -> Logical Operator254/1
  Logical Operator253/1 -> Logical Operator254/8
  Logical Operator252/1 -> Logical Operator254/7
  Logical Operator251/1 -> Logical Operator254/6
  Logical Operator250/1 -> Logical Operator254/5
  Logical Operator241/1 -> Logical Operator254/12
  Logical Operator240/1 -> Logical Operator254/11
  Logical Operator239/1 -> Logical Operator254/10
  Logical Operator255/1 -> Logical Operator254/9
  Logical Operator247/1 -> Logical Operator254/16
  Logical Operator246/1 -> Logical Operator254/15
  Logical Operator245/1 -> Logical Operator254/14
  Logical Operator244/1 -> Logical Operator254/13
  Logical Operator271/1 -> Bus Creator/8
  Logical Operator266/1 -> Logical Operator271/4
  Logical Operator265/1 -> Logical Operator271/3
  Logical Operator260/1 -> Logical Operator271/2
  Logical Operator259/1 -> Logical Operator271/1
  Logical Operator270/1 -> Logical Operator271/8
  Logical Operator269/1 -> Logical Operator271/7
  Logical Operator268/1 -> Logical Operator271/6
  Logical Operator267/1 -> Logical Operator271/5
  Logical Operator258/1 -> Logical Operator271/12
  Logical Operator257/1 -> Logical Operator271/11
  Logical Operator256/1 -> Logical Operator271/10
  Logical Operator272/1 -> Logical Operator271/9
  Logical Operator264/1 -> Logical Operator271/16
  Logical Operator263/1 -> Logical Operator271/15
  Logical Operator262/1 -> Logical Operator271/14
  Logical Operator261/1 -> Logical Operator271/13
  Select_01(1b)/1 -> Logical Operator263/1, Logical Operator246/1, Logical Operator229/1, Logical Operator212/1, Logical Operator195/1, Logical Operator178/1, Logical Operator161/1, Logical Operator144/1
  Select_05(1b)/1 -> Logical Operator257/1, Logical Operator240/1, Logical Operator223/1, Logical Operator206/1, Logical Operator189/1, Logical Operator172/1, Logical Operator155/1, Logical Operator138/1
  Logical Operator254/1 -> Bus Creator/7
  Logical Operator220/1 -> Bus Creator/5
  Logical Operator186/1 -> Bus Creator/3
  Logical Operator152/1 -> Bus Creator/1

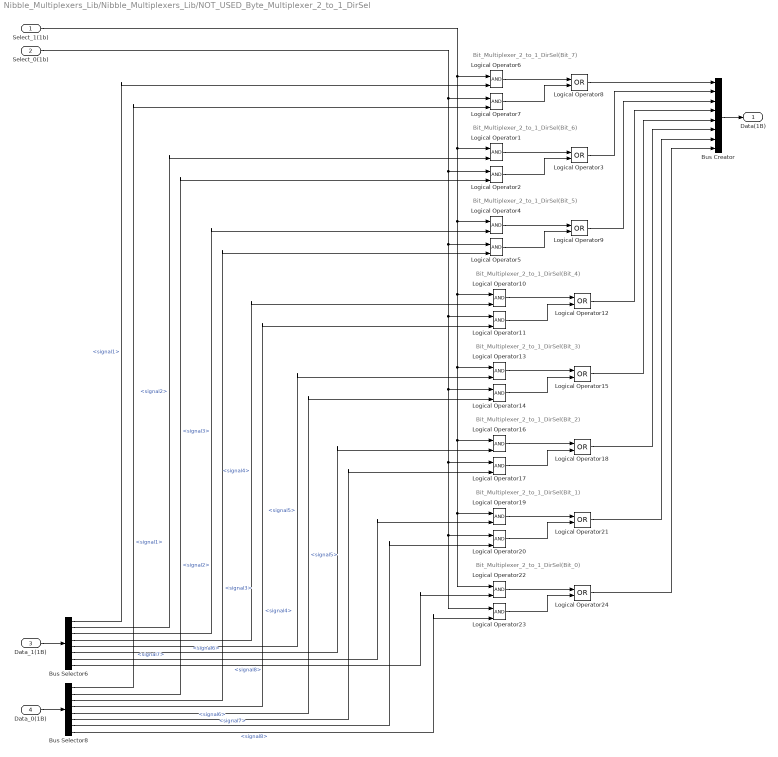
== system Nibble_Multiplexers_Lib/Nibble_Multiplexers_Lib/NOT_USED_Byte_Multiplexer_2_to_1_DirSel ==
  note: Bit_Multiplexer_2_to_1_DirSel(Bit_7)
  note: Bit_Multiplexer_2_to_1_DirSel(Bit_6)
  note: Bit_Multiplexer_2_to_1_DirSel(Bit_5)
  note: Bit_Multiplexer_2_to_1_DirSel(Bit_4)
  note: Bit_Multiplexer_2_to_1_DirSel(Bit_3)
  note: Bit_Multiplexer_2_to_1_DirSel(Bit_2)
  note: Bit_Multiplexer_2_to_1_DirSel(Bit_1)
  note: Bit_Multiplexer_2_to_1_DirSel(Bit_0)
  Select_1(1b) : Inport
  Select_0(1b) : Inport  Port=2
  Data_1(1B) : Inport  Port=3
  Data_0(1B) : Inport  Port=4
  Bus Creator : BusCreator  Inputs=8
  Bus Selector6 : BusSelector  OutputSignals=signal1,signal2,signal3,signal4,signal5,signal6,signal7,signal8
  Bus Selector8 : BusSelector  OutputSignals=signal1,signal2,signal3,signal4,signal5,signal6,signal7,signal8
  Logical Operator{1..2,4..7,10..11,13..14,16..17,19..20,22..23} (16 alike) : Logic  IconShape=distinctive  AllPortsSameDT=off  OutDataTypeStr=boolean
  Logical Operator{3,8..9,12,15,18,21,24} (8 alike) : Logic  Operator=OR  IconShape=distinctive  OutDataTypeStr=boolean
  Data(1B) : Outport
  wires:
  Bus Creator/1 -> Data(1B)/1
  Bus Selector8/8 -> Logical Operator23/2  "<signal8>"
  Bus Selector6/8 -> Logical Operator22/2  "<signal8>"
  Bus Selector8/7 -> Logical Operator20/2  "<signal7>"
  Bus Selector6/7 -> Logical Operator19/2  "<signal7>"
  Bus Selector8/6 -> Logical Operator17/2  "<signal6>"
  Bus Selector6/6 -> Logical Operator16/2  "<signal6>"
  Bus Selector8/5 -> Logical Operator14/2  "<signal5>"
  Bus Selector6/5 -> Logical Operator13/2  "<signal5>"
  Bus Selector8/4 -> Logical Operator11/2  "<signal4>"
  Bus Selector6/4 -> Logical Operator10/2  "<signal4>"
  Bus Selector8/3 -> Logical Operator5/2  "<signal3>"
  Bus Selector6/3 -> Logical Operator4/2  "<signal3>"
  Bus Selector8/2 -> Logical Operator2/2  "<signal2>"
  Bus Selector6/2 -> Logical Operator1/2  "<signal2>"
  Bus Selector8/1 -> Logical Operator7/2  "<signal1>"
  Bus Selector6/1 -> Logical Operator6/2  "<signal1>"
  Select_0(1b)/1 -> Logical Operator20/1, Logical Operator23/1, Logical Operator17/1, Logical Operator14/1, Logical Operator11/1, Logical Operator5/1, Logical Operator2/1, Logical Operator7/1
  Logical Operator3/1 -> Bus Creator/2
  Logical Operator12/1 -> Bus Creator/4
  Logical Operator18/1 -> Bus Creator/6
  Logical Operator24/1 -> Bus Creator/8
  Select_1(1b)/1 -> Logical Operator19/1, Logical Operator22/1, Logical Operator16/1, Logical Operator13/1, Logical Operator10/1, Logical Operator4/1, Logical Operator1/1, Logical Operator6/1
  Logical Operator21/1 -> Bus Creator/7
  Logical Operator15/1 -> Bus Creator/5
  Logical Operator9/1 -> Bus Creator/3
  Logical Operator8/1 -> Bus Creator/1
  Logical Operator7/1 -> Logical Operator8/2
  Logical Operator6/1 -> Logical Operator8/1
  Data_0(1B)/1 -> Bus Selector8/1
  Data_1(1B)/1 -> Bus Selector6/1
  Logical Operator2/1 -> Logical Operator3/2
  Logical Operator1/1 -> Logical Operator3/1
  Logical Operator5/1 -> Logical Operator9/2
  Logical Operator4/1 -> Logical Operator9/1
  Logical Operator11/1 -> Logical Operator12/2
  Logical Operator10/1 -> Logical Operator12/1
  Logical Operator14/1 -> Logical Operator15/2
  Logical Operator13/1 -> Logical Operator15/1
  Logical Operator17/1 -> Logical Operator18/2
  Logical Operator16/1 -> Logical Operator18/1
  Logical Operator20/1 -> Logical Operator21/2
  Logical Operator19/1 -> Logical Operator21/1
  Logical Operator23/1 -> Logical Operator24/2
  Logical Operator22/1 -> Logical Operator24/1

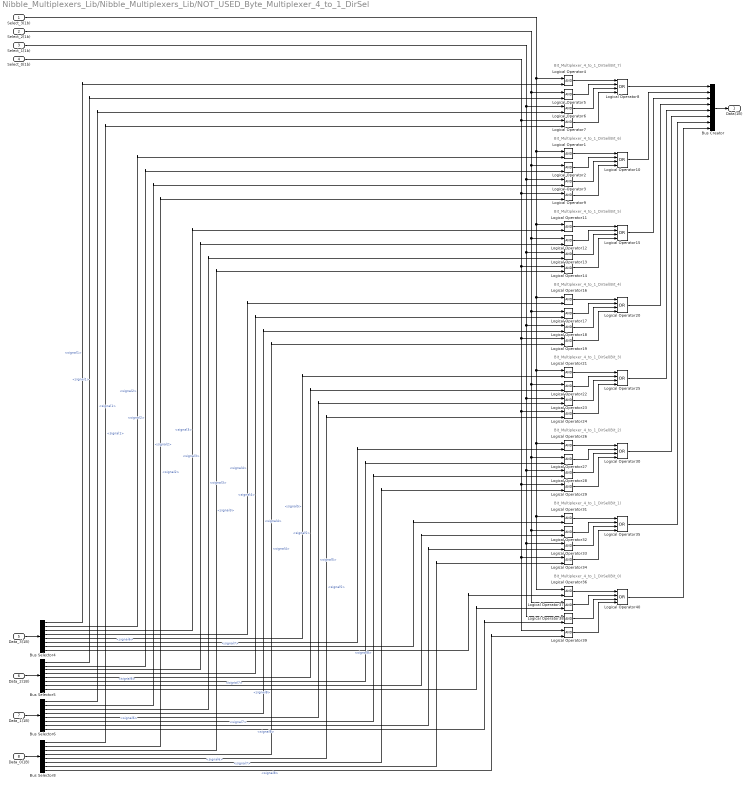
== system Nibble_Multiplexers_Lib/Nibble_Multiplexers_Lib/NOT_USED_Byte_Multiplexer_4_to_1_DirSel ==
  note: Bit_Multiplexer_4_to_1_DirSel(Bit_7)
  note: Bit_Multiplexer_4_to_1_DirSel(Bit_6)
  note: Bit_Multiplexer_4_to_1_DirSel(Bit_5)
  note: Bit_Multiplexer_4_to_1_DirSel(Bit_4)
  note: Bit_Multiplexer_4_to_1_DirSel(Bit_3)
  note: Bit_Multiplexer_4_to_1_DirSel(Bit_2)
  note: Bit_Multiplexer_4_to_1_DirSel(Bit_1)
  note: Bit_Multiplexer_4_to_1_DirSel(Bit_0)
  Select_3(1b) : Inport
  Select_2(1b) : Inport  Port=2
  Select_1(1b) : Inport  Port=3
  Select_0(1b) : Inport  Port=4
  Data_3(1B) : Inport  Port=5
  Data_2(1B) : Inport  Port=6
  Data_1(1B) : Inport  Port=7
  Data_0(1B) : Inport  Port=8
  Bus Creator : BusCreator  Inputs=8
  Bus Selector{4..6,8} (4 alike) : BusSelector  OutputSignals=signal1,signal2,signal3,signal4,signal5,signal6,signal7,signal8
  Logical Operator{1..7,9,11..14,16..19,21..24,26..29,31..34,36..39} (32 alike) : Logic  IconShape=distinctive  AllPortsSameDT=off  OutDataTypeStr=boolean
  Logical Operator{8,10,15,20,25,30,35,40} (8 alike) : Logic  Operator=OR  Inputs=4  IconShape=distinctive  OutDataTypeStr=boolean
  Data(1B) : Outport
  wires:
  Bus Creator/1 -> Data(1B)/1
  Bus Selector8/8 -> Logical Operator39/2  "<signal8>"
  Bus Selector6/8 -> Logical Operator38/2  "<signal8>"
  Bus Selector5/8 -> Logical Operator37/2  "<signal8>"
  Bus Selector4/8 -> Logical Operator36/2  "<signal8>"
  Bus Selector8/7 -> Logical Operator34/2  "<signal7>"
  Bus Selector6/7 -> Logical Operator33/2  "<signal7>"
  Bus Selector5/7 -> Logical Operator32/2  "<signal7>"
  Bus Selector4/7 -> Logical Operator31/2  "<signal7>"
  Bus Selector8/6 -> Logical Operator29/2  "<signal6>"
  Bus Selector6/6 -> Logical Operator28/2  "<signal6>"
  Bus Selector5/6 -> Logical Operator27/2  "<signal6>"
  Bus Selector4/6 -> Logical Operator26/2  "<signal6>"
  Bus Selector8/5 -> Logical Operator24/2  "<signal5>"
  Bus Selector6/5 -> Logical Operator23/2  "<signal5>"
  Bus Selector5/5 -> Logical Operator22/2  "<signal5>"
  Bus Selector4/5 -> Logical Operator21/2  "<signal5>"
  Bus Selector8/4 -> Logical Operator19/2  "<signal4>"
  Bus Selector6/4 -> Logical Operator18/2  "<signal4>"
  Bus Selector5/4 -> Logical Operator17/2  "<signal4>"
  Bus Selector4/4 -> Logical Operator16/2  "<signal4>"
  Bus Selector8/3 -> Logical Operator14/2  "<signal3>"
  Bus Selector6/3 -> Logical Operator13/2  "<signal3>"
  Bus Selector5/3 -> Logical Operator12/2  "<signal3>"
  Bus Selector4/3 -> Logical Operator11/2  "<signal3>"
  Bus Selector8/2 -> Logical Operator9/2  "<signal2>"
  Bus Selector6/2 -> Logical Operator3/2  "<signal2>"
  Bus Selector5/2 -> Logical Operator2/2  "<signal2>"
  Bus Selector4/2 -> Logical Operator1/2  "<signal2>"
  Bus Selector8/1 -> Logical Operator7/2  "<signal1>"
  Bus Selector6/1 -> Logical Operator6/2  "<signal1>"
  Bus Selector5/1 -> Logical Operator5/2  "<signal1>"
  Bus Selector4/1 -> Logical Operator4/2  "<signal1>"
  Select_3(1b)/1 -> Logical Operator16/1, Logical Operator21/1, Logical Operator26/1, Logical Operator36/1, Logical Operator31/1, Logical Operator11/1, Logical Operator1/1, Logical Operator4/1
  Select_2(1b)/1 -> Logical Operator17/1, Logical Operator22/1, Logical Operator27/1, Logical Operator37/1, Logical Operator32/1, Logical Operator12/1, Logical Operator2/1, Logical Operator5/1
  Select_0(1b)/1 -> Logical Operator19/1, Logical Operator24/1, Logical Operator29/1, Logical Operator39/1, Logical Operator34/1, Logical Operator14/1, Logical Operator9/1, Logical Operator7/1
  Logical Operator10/1 -> Bus Creator/2
  Logical Operator20/1 -> Bus Creator/4
  Logical Operator30/1 -> Bus Creator/6
  Logical Operator40/1 -> Bus Creator/8
  Select_1(1b)/1 -> Logical Operator18/1, Logical Operator23/1, Logical Operator28/1, Logical Operator38/1, Logical Operator33/1, Logical Operator13/1, Logical Operator3/1, Logical Operator6/1
  Logical Operator35/1 -> Bus Creator/7
  Logical Operator25/1 -> Bus Creator/5
  Logical Operator15/1 -> Bus Creator/3
  Logical Operator8/1 -> Bus Creator/1
  Logical Operator7/1 -> Logical Operator8/4
  Logical Operator6/1 -> Logical Operator8/3
  Logical Operator5/1 -> Logical Operator8/2
  Logical Operator4/1 -> Logical Operator8/1
  Data_0(1B)/1 -> Bus Selector8/1
  Data_1(1B)/1 -> Bus Selector6/1
  Data_2(1B)/1 -> Bus Selector5/1
  Data_3(1B)/1 -> Bus Selector4/1
  Logical Operator9/1 -> Logical Operator10/4
  Logical Operator3/1 -> Logical Operator10/3
  Logical Operator2/1 -> Logical Operator10/2
  Logical Operator1/1 -> Logical Operator10/1
  Logical Operator14/1 -> Logical Operator15/4
  Logical Operator13/1 -> Logical Operator15/3
  Logical Operator12/1 -> Logical Operator15/2
  Logical Operator11/1 -> Logical Operator15/1
  Logical Operator19/1 -> Logical Operator20/4
  Logical Operator18/1 -> Logical Operator20/3
  Logical Operator17/1 -> Logical Operator20/2
  Logical Operator16/1 -> Logical Operator20/1
  Logical Operator24/1 -> Logical Operator25/4
  Logical Operator23/1 -> Logical Operator25/3
  Logical Operator22/1 -> Logical Operator25/2
  Logical Operator21/1 -> Logical Operator25/1
  Logical Operator29/1 -> Logical Operator30/4
  Logical Operator28/1 -> Logical Operator30/3
  Logical Operator27/1 -> Logical Operator30/2
  Logical Operator26/1 -> Logical Operator30/1
  Logical Operator34/1 -> Logical Operator35/4
  Logical Operator33/1 -> Logical Operator35/3
  Logical Operator32/1 -> Logical Operator35/2
  Logical Operator31/1 -> Logical Operator35/1
  Logical Operator39/1 -> Logical Operator40/4
  Logical Operator38/1 -> Logical Operator40/3
  Logical Operator37/1 -> Logical Operator40/2
  Logical Operator36/1 -> Logical Operator40/1
